simulink model "gm_hdl_model_fixed"  (R2024a)
settings: Solver=FixedStepDiscrete  StartTime=0.0  StopTime=SIM_TIME  RelTol=1e-3
model workspace (MAT data in the model file):
  HDLVAXIManagerConfig = hdlverifier.internal.AXIMaster.ConfigParams
undefined symbols (not defined in the file or in its folder): a, b, BUFFER_LEN, c, SAMPLING_FREQ, signal_1
libraries: hdlsllib x38, simulink_extras x4, simulink x2, dspsrcs4 x1, dsphdlxfrm2 x1
(part 1 of 3)
settings Model: SimulationMode=accelerator  Creator=Jan Rosa  LastModifiedBy=Jan Rosa
settings OptimizationCC: BlockReduction=off  ConditionallyExecuteInputs=off  DefaultParameterBehavior=Inlined  InheritOutputTypeSmallerThanSingle=on
settings DebuggingCC: SignalRangeChecking=warning  AlgebraicLoopMsg=error  SolverPrmCheckMsg=warning  InheritedTsInSrcMsg=none  SingleTaskRateTransMsg=error  UnderSpecifiedDataTypeMsg=warning  UnconnectedInputMsg=error  UnconnectedOutputMsg=error  UnconnectedLineMsg=error  ModelReferenceVersionMismatchMessage=warning  ModelReferenceIOMismatchMessage=warning  ModelReferenceNoExplicitFinalValueMsg=warning  StateNameClashWarn=warning
settings HardwareCC: ProdBitPerPointer=32  ProdBitPerSizeT=32  ProdBitPerPtrDiffT=32  ProdLargestAtomicFloat=None  ProdIntDivRoundTo=Undefined  ProdEndianess=Unspecified  ProdWordSize=32  ProdHWDeviceType=ASIC/FPGA->ASIC/FPGA  TargetBitPerPointer=64  TargetBitPerSizeT=64  TargetBitPerPtrDiffT=64  TargetLongLongMode=on  TargetIntDivRoundTo=Zero  TargetEndianess=LittleEndian  TargetWordSize=64  TargetHWDeviceType=Custom Processor->MATLAB Host Computer  ProdEqTarget=off
settings ModelReferenceCC: EnableRefExpFcnMdlSchedulingChecks=on  EnableParallelModelReferenceBuilds=on

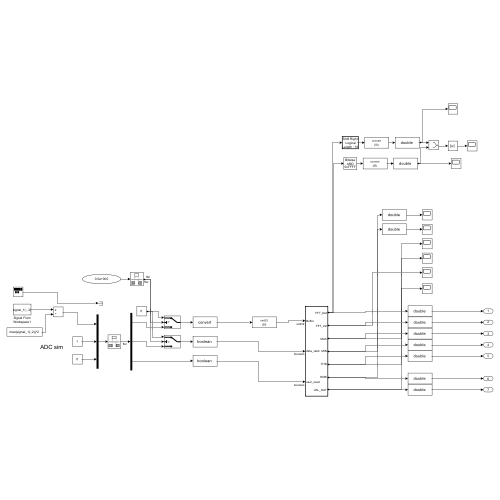
[thumbnail: Simulink's stored preview of the top-level diagram]
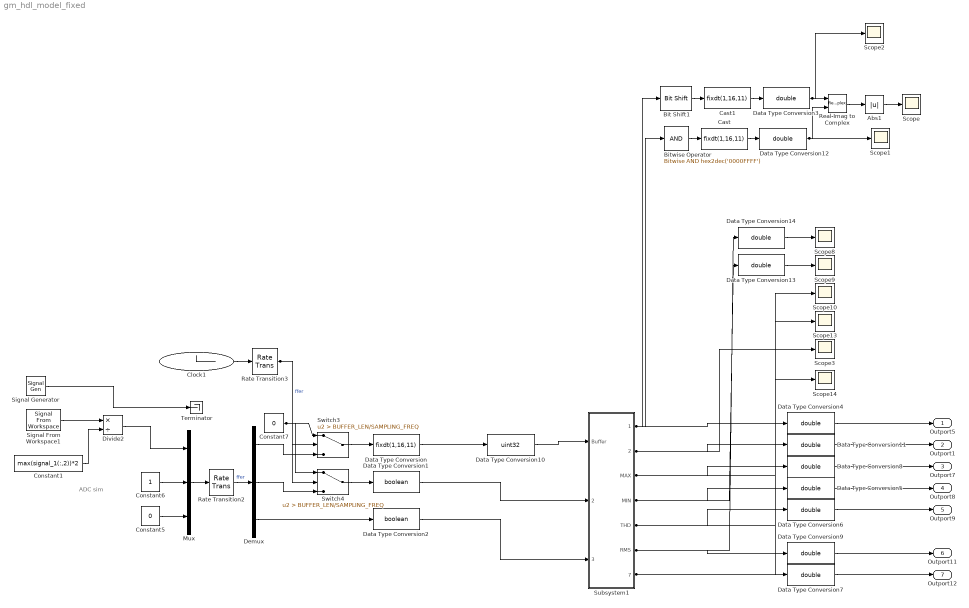
== system gm_hdl_model_fixed ==
  note: ADC sim
  Abs1 : Abs  SaturateOnIntegerOverflow=off
  Bit Shift1 : hdlsllib/Logic and Bit Operations/Bit Shift  mode=Shift Right Logical  N=16
  Bitwise Operator : simulink/Logic and Bit Operations/Bitwise Operator  logicop=AND  UseBitMask=on  BitMask=hex2dec('0000FFFF')  BitMaskRealWorld=Stored Integer
  Cast : DataTypeConversion  OutDataTypeStr=fixdt(1,16,11)  ConvertRealWorld=Stored Integer (SI)  SaturateOnIntegerOverflow=off  RndMeth=Floor
  Cast1 : DataTypeConversion  OutDataTypeStr=fixdt(1,16,11)  ConvertRealWorld=Stored Integer (SI)  SaturateOnIntegerOverflow=off  RndMeth=Floor
  Clock1 : Clock
  Constant1 : Constant  Value=max(signal_1(:,2))*2
  Constant5 : Constant  Value=0
  Constant6 : Constant
  Constant7 : Constant  Value=0  SampleTime=1/SAMPLING_FREQ
  Data Type Conversion : DataTypeConversion  OutDataTypeStr=fixdt(1,16,11)  SaturateOnIntegerOverflow=off  RndMeth=Floor  LockScale=on
  Data Type Conversion1 : DataTypeConversion  OutDataTypeStr=boolean  SaturateOnIntegerOverflow=off  RndMeth=Floor  LockScale=on
  Data Type Conversion10 : DataTypeConversion  OutDataTypeStr=uint32  ConvertRealWorld=Stored Integer (SI)  SaturateOnIntegerOverflow=off  RndMeth=Floor
  Data Type Conversion{3..9,11..14} (11 alike) : DataTypeConversion  OutDataTypeStr=double  SaturateOnIntegerOverflow=off  RndMeth=Floor
  Data Type Conversion2 : DataTypeConversion  OutDataTypeStr=boolean  SaturateOnIntegerOverflow=off  RndMeth=Floor  LockScale=on
  Demux : Demux  Outputs=3
  Divide2 : Product  Inputs=*/
  Mux : Mux  Inputs=3
  Rate Transition2 : RateTransition  Integrity=off  Deterministic=off  OutPortSampleTime=1/SAMPLING_FREQ
  Rate Transition3 : RateTransition  Integrity=off  Deterministic=off  OutPortSampleTime=1/SAMPLING_FREQ
  Real-Imag to Complex : RealImagToComplex
  Scope{,1..3,8..10,13..14} (9 alike) : Scope
  Signal Generator : SignalGenerator  WaveForm=square  Amplitude=0.49999  Frequency=SAMPLING_FREQ/(16*16)
  Signal From Workspace1 : dspsrcs4/Signal From Workspace  X=signal_1(:, 2)  Ts=1/SAMPLING_FREQ  nsamps=1  OutputAfterFinalValue=Cyclic repetition  ignoreOrWarnInputAndFrameLengths=off  OutputFrames=off
  Subsystem1 : Subsystem  TreatAsAtomicUnit=on
  Switch3 : Switch  Criteria=u2 > Threshold  Threshold=BUFFER_LEN/SAMPLING_FREQ  SaturateOnIntegerOverflow=off  InputSameDT=off
  Switch4 : Switch  Criteria=u2 > Threshold  Threshold=BUFFER_LEN/SAMPLING_FREQ  SaturateOnIntegerOverflow=off  InputSameDT=off
  Terminator : Terminator
  Outport5 : Outport
  Outport1 : Outport  Port=2
  Outport7 : Outport  Port=3
  Outport8 : Outport  Port=4
  Outport9 : Outport  Port=5
  Outport11 : Outport  Port=6
  Outport12 : Outport  Port=7
  wires:
  Data Type Conversion10/1 -> Subsystem1/1(Buffer)
  Signal Generator/1 -> Terminator/1
  Divide2/1 -> Mux/1
  Subsystem1/2(FFT_Val) -> Data Type Conversion11/1, Scope3/1
  Data Type Conversion/1 -> Data Type Conversion10/1
  Data Type Conversion1/1 -> Subsystem1/2(data_valid)
  Data Type Conversion2/1 -> Subsystem1/3(user_reset)
  Switch4/1 -> Data Type Conversion1/1
  Data Type Conversion13/1 -> Scope9/1
  Data Type Conversion14/1 -> Scope8/1
  Cast1/1 -> Data Type Conversion3/1
  Cast/1 -> Data Type Conversion12/1
  Data Type Conversion12/1 -> Real-Imag to Complex/2, Scope1/1
  Bitwise Operator/1 -> Cast/1
  Bit Shift1/1 -> Cast1/1
  Real-Imag to Complex/1 -> Abs1/1
  Data Type Conversion3/1 -> Real-Imag to Complex/1, Scope2/1
  Data Type Conversion11/1 -> Outport1/1
  Data Type Conversion9/1 -> Outport11/1
  Data Type Conversion7/1 -> Outport12/1
  Data Type Conversion6/1 -> Outport9/1
  Data Type Conversion5/1 -> Outport8/1
  Data Type Conversion8/1 -> Outport7/1
  Data Type Conversion4/1 -> Outport5/1
  Subsystem1/6(RMS) -> Data Type Conversion14/1, Data Type Conversion9/1
  Constant1/1 -> Divide2/2
  Constant6/1 -> Mux/2
  Signal From Workspace1/1 -> Divide2/1
  Constant5/1 -> Mux/3
  Rate Transition2/1 -> Demux/1  "ffer"
  Abs1/1 -> Scope/1
  Subsystem1/4(MIN) -> Data Type Conversion13/1, Data Type Conversion5/1
  Mux/1 -> Rate Transition2/1
  Demux/1 -> Switch3/3
  Switch3/1 -> Data Type Conversion/1
  Subsystem1/5(THD) -> Scope13/1, Data Type Conversion6/1
  Demux/3 -> Data Type Conversion2/1
  Clock1/1 -> Rate Transition3/1
  Demux/2 -> Switch4/3
  Subsystem1/3(MAX) -> Scope10/1, Data Type Conversion8/1
  Subsystem1/7(VAL_OUT) -> Scope14/1, Data Type Conversion7/1
  Rate Transition3/1 -> Switch3/2, Switch4/2  "ffer"
  Constant7/1 -> Switch3/1, Switch4/1
  Subsystem1/1(FFT_Dat) -> Bit Shift1/1, Bitwise Operator/1, Data Type Conversion4/1

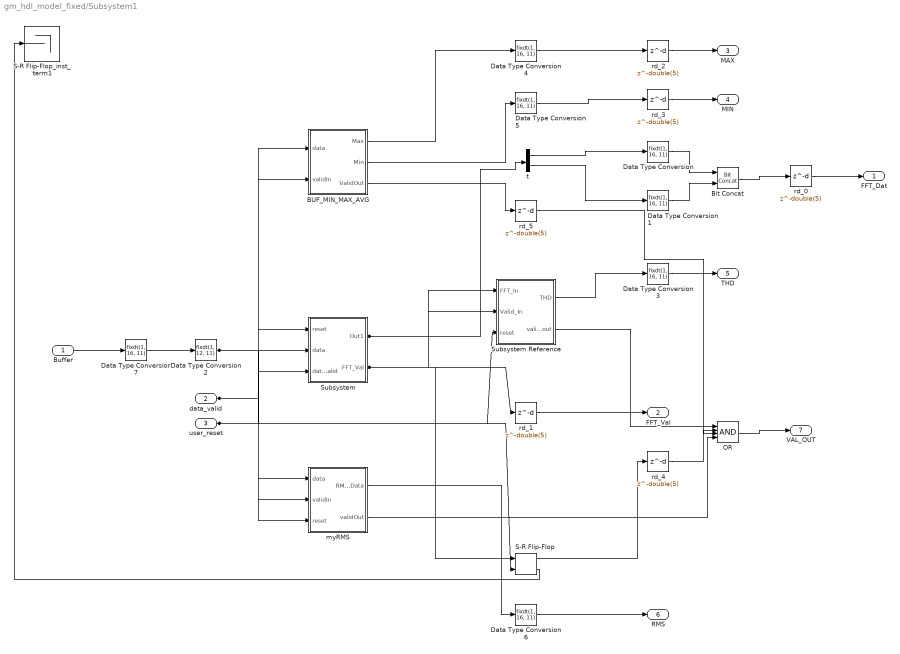
== system gm_hdl_model_fixed/Subsystem1 ==
  Buffer : Inport  OutDataTypeStr=uint32  PortDimensions=1  SampleTime=1e-08
  data_valid : Inport  Port=2  OutDataTypeStr=boolean  PortDimensions=1  SampleTime=1e-08
  user_reset : Inport  Port=3  OutDataTypeStr=boolean  PortDimensions=1  SampleTime=1e-08
  BUF_MIN_MAX_AVG : Subsystem
  Bit Concat : hdlsllib/Logic and Bit Operations/Bit Concat  numInputs=2
  Data Type Conversion{,1,3..6} (6 alike) : DataTypeConversion  OutDataTypeStr=fixdt(1, 16, 11)  SampleTime=1e-08  SaturateOnIntegerOverflow=off  RndMeth=Floor
  Data Type Conversion2 : DataTypeConversion  OutDataTypeStr=fixdt(1, 12, 11)  SampleTime=1e-08  SaturateOnIntegerOverflow=off  RndMeth=Floor
  Data Type Conversion7 : DataTypeConversion  OutDataTypeStr=fixdt(1, 16, 11)  ConvertRealWorld=Stored Integer (SI)  SampleTime=1e-08  SaturateOnIntegerOverflow=off  RndMeth=Floor
  OR : Logic  Inputs=4  AllPortsSameDT=off  OutDataTypeStr=boolean  SampleTime=1e-08
  S-R Flip-Flop : simulink_extras/Flip Flops/S-R Flip-Flop  initial_condition=0
  S-R Flip-Flop_inst_term1 : Terminator
  Subsystem : Subsystem
  Subsystem Reference : Subsystem
  myRMS : Subsystem
  rd_{0..5} (6 alike) : Delay  DelayLength=double(5)  InitialCondition=0  SampleTime=1e-08
  t : Demux  Outputs=2
  FFT_Dat : Outport  SampleTime=1e-08
  FFT_Val : Outport  Port=2  SampleTime=1e-08
  MAX : Outport  Port=3  SampleTime=1e-08
  MIN : Outport  Port=4  SampleTime=1e-08
  THD : Outport  Port=5  SampleTime=1e-08
  RMS : Outport  Port=6  SampleTime=1e-08
  VAL_OUT : Outport  Port=7  SampleTime=1e-08
  wires:
  Buffer/1 -> Data Type Conversion7/1
  data_valid/1 -> Subsystem/3(data_valid), myRMS/2(validIn), BUF_MIN_MAX_AVG/2(validIn)
  user_reset/1 -> Subsystem Reference/3(reset), Subsystem/1(reset), myRMS/3(reset), S-R Flip-Flop/2
  BUF_MIN_MAX_AVG/1(Max) -> Data Type Conversion4/1
  BUF_MIN_MAX_AVG/2(Min) -> Data Type Conversion5/1
  Data Type Conversion/1 -> Bit Concat/1
  Data Type Conversion1/1 -> Bit Concat/2
  Data Type Conversion2/1 -> Subsystem/2(data), BUF_MIN_MAX_AVG/1(data), myRMS/1(data)
  Data Type Conversion3/1 -> THD/1
  Data Type Conversion6/1 -> RMS/1
  Data Type Conversion7/1 -> Data Type Conversion2/1
  OR/1 -> VAL_OUT/1
  S-R Flip-Flop/2 -> S-R Flip-Flop_inst_term1/1
  Subsystem/1(Out1) -> t/1, Subsystem Reference/1(FFT_In)
  Subsystem Reference/1(THD) -> Data Type Conversion3/1
  Subsystem Reference/2(valid_out) -> OR/1
  myRMS/1(RMS_Data) -> Data Type Conversion6/1
  myRMS/2(validOut) -> OR/4
  t/1 -> Data Type Conversion/1
  t/2 -> Data Type Conversion1/1
  S-R Flip-Flop/1 -> rd_4/1
  BUF_MIN_MAX_AVG/3(ValidOut) -> rd_5/1
  Bit Concat/1 -> rd_0/1
  Subsystem/2(FFT_Val) -> rd_1/1, Subsystem Reference/2(Valid_In), S-R Flip-Flop/1
  Data Type Conversion4/1 -> rd_2/1
  Data Type Conversion5/1 -> rd_3/1
  rd_5/1 -> OR/3
  rd_1/1 -> FFT_Val/1
  rd_0/1 -> FFT_Dat/1
  rd_2/1 -> MAX/1
  rd_3/1 -> MIN/1
  rd_4/1 -> OR/2

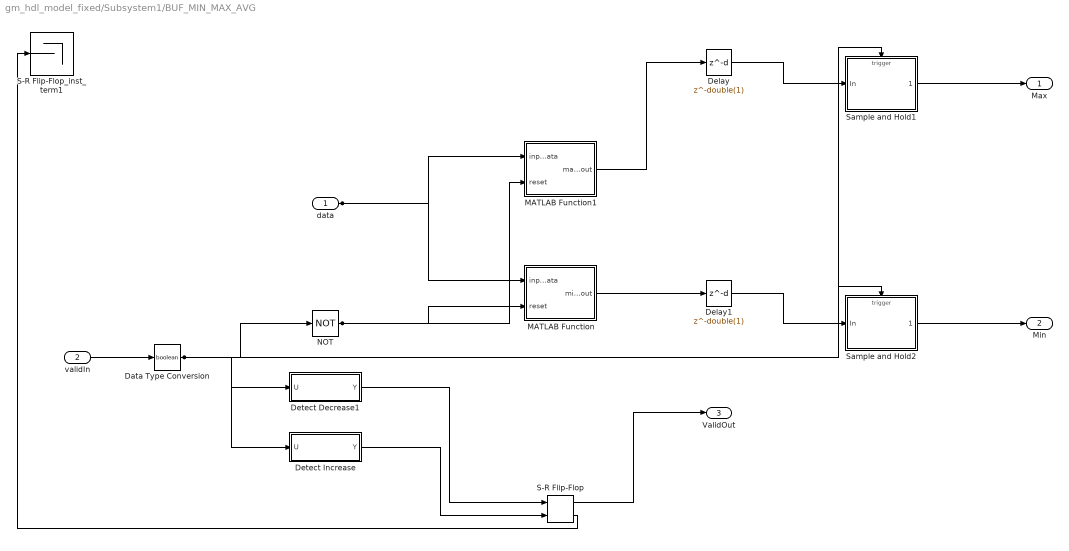
== system gm_hdl_model_fixed/Subsystem1/BUF_MIN_MAX_AVG ==
  data : Inport  OutDataTypeStr=fixdt(1, 12, 11)  PortDimensions=1  SampleTime=1e-08
  validIn : Inport  Port=2  OutDataTypeStr=boolean  PortDimensions=1  SampleTime=1e-08
  Data Type Conversion : DataTypeConversion  OutDataTypeStr=boolean
  Delay : Delay  DelayLength=double(1)  InitialCondition=0  SampleTime=1e-08
  Delay1 : Delay  DelayLength=double(1)  InitialCondition=0  SampleTime=1e-08
  Detect Decrease1 : Subsystem  mask(Detect Decrease){vinit=double(0), InputProcessing=Elements as channels (sample based), OutDataTypeStr=boolean}
      mask prompts: vinit "Simulink:masks:InitialCondition_MP"; InputProcessing "Simulink:masks:InputProcessing_MP"; OutDataTypeStr "Simulink:masks:OutputDataType_MP"
      mask help: Simulink:masks:DetectDecrease_MD
      mask init:
      | InputProcessing = 'Elements as channels (sample based)';
      | OutDataTypeStr = 'boolean';
      | vinit = double(0);
      mask TypeOptions InputProcessing: Simulink:masks:ColumnsAsChannelsFrameBased | Simulink:masks:ElementsAsChannelsSampleBased
      mask TypeOptions OutDataTypeStr: Simulink:masks:uint8 | Simulink:masks:boolean
      mask Display: fprintf('U < U/z')
  Detect Increase : Subsystem  mask(Detect Increase){vinit=double(0), InputProcessing=Elements as channels (sample based), OutDataTypeStr=boolean}
      mask prompts: vinit "Simulink:masks:InitialCondition_MP"; InputProcessing "Simulink:masks:InputProcessing_MP"; OutDataTypeStr "Simulink:masks:OutputDataType_MP"
      mask help: Simulink:masks:DetectIncrease_MD
      mask init:
      | InputProcessing = 'Elements as channels (sample based)';
      | OutDataTypeStr = 'boolean';
      | vinit = double(0);
      mask TypeOptions InputProcessing: Simulink:masks:ColumnsAsChannelsFrameBased | Simulink:masks:ElementsAsChannelsSampleBased
      mask TypeOptions OutDataTypeStr: Simulink:masks:uint8 | Simulink:masks:boolean
      mask Display: fprintf('U > U/z')
  MATLAB Function : Subsystem
  MATLAB Function1 : Subsystem
  NOT : Logic  Operator=NOT  Inputs=1  AllPortsSameDT=off  OutDataTypeStr=boolean  SampleTime=1e-08
  S-R Flip-Flop : simulink_extras/Flip Flops/S-R Flip-Flop  initial_condition=0
  S-R Flip-Flop_inst_term1 : Terminator
  Sample and Hold1 : Subsystem  mask(Sample and Hold){trig=Falling edge, initCond=double(0), latchinput=off}
      mask prompts: trig "dsp:DSPSignalOperationsBlockDialog:TriggerType_MP"; initCond "dsp:DSPSignalOperationsBlockDialog:InitialCondition_MP"; latchinput "dsp:DSPSignalOperationsBlockDialog:LatchInput_MP"
      mask help: dsp:DSPSignalOperationsBlockDialog:SampleAndHold_MaskDesc
      mask init:
      | initCond = double(0);
      | latchinput = double(0);
      | s = 'falling';
      | trig = double(2);
      mask Help: eval('blocksethelp');
      mask TypeOptions trig: dsp:DSPSignalOperationsBlockDialog:RisingEdge_MP | dsp:DSPSignalOperationsBlockDialog:FallingEdge_MP | dsp:DSPSignalOperationsBlockDialog:EitherEdge_MP
      mask Display: disp('S/H')
  Sample and Hold2 : Subsystem  mask(Sample and Hold){trig=Falling edge, initCond=double(0), latchinput=off}
      mask prompts: trig "dsp:DSPSignalOperationsBlockDialog:TriggerType_MP"; initCond "dsp:DSPSignalOperationsBlockDialog:InitialCondition_MP"; latchinput "dsp:DSPSignalOperationsBlockDialog:LatchInput_MP"
      mask help: dsp:DSPSignalOperationsBlockDialog:SampleAndHold_MaskDesc
      mask init:
      | initCond = double(0);
      | latchinput = double(0);
      | s = 'falling';
      | trig = double(2);
      mask Help: eval('blocksethelp');
      mask TypeOptions trig: dsp:DSPSignalOperationsBlockDialog:RisingEdge_MP | dsp:DSPSignalOperationsBlockDialog:FallingEdge_MP | dsp:DSPSignalOperationsBlockDialog:EitherEdge_MP
      mask Display: disp('S/H')
  Max : Outport  SampleTime=1e-08
  Min : Outport  Port=2  SampleTime=1e-08
  ValidOut : Outport  Port=3  SampleTime=1e-08
  wires:
  data/1 -> MATLAB Function1/1(input_data), MATLAB Function/1(input_data)
  validIn/1 -> Data Type Conversion/1
  Data Type Conversion/1 -> NOT/1, Detect Increase/1(U), Detect Decrease1/1(U), Sample and Hold1/Trigger, Sample and Hold2/Trigger
  Delay/1 -> Sample and Hold1/1(In)
  Delay1/1 -> Sample and Hold2/1(In)
  Detect Decrease1/1(Y) -> S-R Flip-Flop/1
  Detect Increase/1(Y) -> S-R Flip-Flop/2
  MATLAB Function/1(min_out) -> Delay1/1
  MATLAB Function1/1(max_out) -> Delay/1
  NOT/1 -> MATLAB Function1/2(reset), MATLAB Function/2(reset)
  S-R Flip-Flop/1 -> ValidOut/1
  S-R Flip-Flop/2 -> S-R Flip-Flop_inst_term1/1
  Sample and Hold1/1(" ") -> Max/1
  Sample and Hold2/1(" ") -> Min/1

== system gm_hdl_model_fixed/Subsystem1/Subsystem ==
  note: Divide by FFT length shift
  reset : Inport  OutDataTypeStr=boolean  PortDimensions=1  SampleTime=1e-08
  data : Inport  Port=2  OutDataTypeStr=fixdt(1, 12, 11)  PortDimensions=1  SampleTime=1e-08
  data_valid : Inport  Port=3  OutDataTypeStr=boolean  PortDimensions=1  SampleTime=1e-08
  Bit Shift : hdlsllib/Logic and Bit Operations/Bit Shift  mode=Shift Right Arithmetic  N=double(11)
  Complex to Real-Imag : ComplexToRealImag  SampleTime=1e-08
  Data Type Conversion : DataTypeConversion  OutDataTypeStr=fixdt(1, 12, 11)  SampleTime=1e-08  SaturateOnIntegerOverflow=off  RndMeth=Floor
  FFT : dsphdlxfrm2/FFT  Architecture=Streaming Radix 2^2  FFTLengthSource=Property  FFTLength=BUFFER_LEN  FFTLengthMax=1024  ComplexMultiplication=Use 4 multipliers and 2 adders  BitReversedOutput=off  BitReversedInput=off  Normalize=off  SimulateUsing=Code generation  RoundingMethod=Floor  ResetInputPort=on  StartOutputPort=off  EndOutputPort=off
  mux : Mux  Inputs=2
  Out1 : Outport  SampleTime=1e-08
  FFT_Val : Outport  Port=2  SampleTime=1e-08
  wires:
  reset/1 -> FFT/3
  data/1 -> FFT/1
  data_valid/1 -> FFT/2
  Bit Shift/1 -> Data Type Conversion/1
  Complex to Real-Imag/1 -> mux/1
  Complex to Real-Imag/2 -> mux/2
  Data Type Conversion/1 -> Out1/1
  FFT/1 -> Complex to Real-Imag/1
  FFT/2 -> FFT_Val/1
  mux/1 -> Bit Shift/1

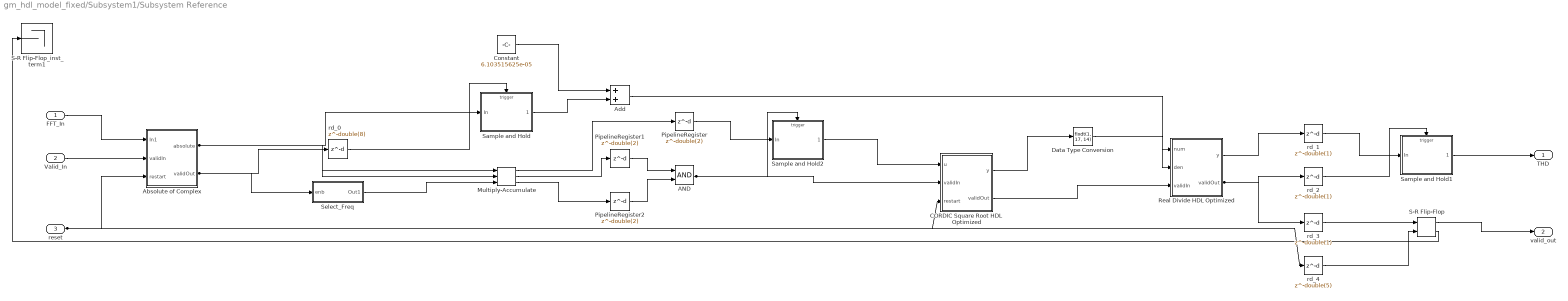
== system gm_hdl_model_fixed/Subsystem1/Subsystem Reference ==
  FFT_In : Inport  OutDataTypeStr=fixdt(1, 12, 11)  PortDimensions=[2]  SampleTime=1e-08
  Valid_In : Inport  Port=2  OutDataTypeStr=boolean  PortDimensions=1  SampleTime=1e-08
  reset : Inport  Port=3  OutDataTypeStr=boolean  PortDimensions=1  SampleTime=1e-08
  AND : Logic  AllPortsSameDT=off  OutDataTypeStr=boolean  SampleTime=1e-08
  Absolute of Complex : Subsystem
  Add : Sum  OutDataTypeStr=fixdt(1, 17, 14)  AccumDataTypeStr=fixdt(1, 17, 14)  SampleTime=1e-08
  CORDIC Square Root HDL Optimized : Subsystem  mask(CORDIC Square Root HDL Optimized){autoMaximumShiftVal=on, maximumShiftValue=double(10), nIterPerReg=double(1)}
      mask prompts: autoMaximumShiftVal "fixed:emblib:AutoCORDICMaxShiftValue"; maximumShiftValue "fixed:emblib:CORDICMaxShiftValue"; nIterPerReg "fixed:emblib:NumberOfIterationsPerReg"
      mask help: fixed:emblib:CORDICSquareRootHDLFullDescription
      mask Help: eval('embblk.embhelp(gcb)')
      mask Callback autoMaximumShiftVal:
      | autoMaxShiftVal = get_param(gcb,'autoMaximumShiftVal');
      | if strcmp(autoMaxShiftVal,'on')
      |     set_param(gcb,'MaskVisibilities',{'on','off','on'});
      | else
      |     set_param(gcb,'MaskVisibilities',{'on','on','on'});
      | end
      mask Display: disp('CORDIC Square Root\nHDL Optimized')
  Constant : Constant  Value=6.103515625e-05  OutDataTypeStr=fixdt(1, 16, 14)  SampleTime=1e-08
  Data Type Conversion : DataTypeConversion  OutDataTypeStr=fixdt(1, 17, 14)  SampleTime=1e-08  SaturateOnIntegerOverflow=off  RndMeth=Floor
  Multiply-Accumulate : hdlsllib/HDL Operations/Multiply-Accumulate  opMode=Streaming - using Number of Samples  initValueSetting=Dialog  initValue=0  initValueSetting2=Dialog  initValue2=0  initValueSetting3=Dialog  initValue3=0  num_samples=1015  RndMeth2=Floor  RndMeth3=Floor  datatype2=Inherit: Inherit via back propagation  datatype3=fixdt(1, 22, 20)  validOut=on  endInandOut=on  startOut=on  countOut=off  dim=-1  DoSatur=off  parallel=off
  PipelineRegister : Delay  DelayLength=double(2)  InitialCondition=0  SampleTime=1e-08
  PipelineRegister1 : Delay  DelayLength=double(2)  InitialCondition=0  SampleTime=1e-08
  PipelineRegister2 : Delay  DelayLength=double(2)  InitialCondition=0  SampleTime=1e-08
  Real Divide HDL Optimized : Subsystem  mask(Real Divide HDL Optimized){OutputType=fixdt(1,18,10)}
      mask prompts: OutputType "fixed:emblib:OutputPrototype"
      mask help: fixed:emblib:RealDivideFullDescription
      mask Help: eval('embblk.embhelp(gcb)')
      mask Display:
      | text(0.5,0.6,'den ~= 0','texmode','on','HorizontalAlignment','center')
      | text(0.5,0.4,'y = num/den','texmode','on','HorizontalAlignment','center')
  S-R Flip-Flop : simulink_extras/Flip Flops/S-R Flip-Flop  initial_condition=0
  S-R Flip-Flop_inst_term1 : Terminator
  Sample and Hold : Subsystem  mask(Sample and Hold){trig=Rising edge, initCond=double(0), latchinput=off}
      mask prompts: trig "dsp:DSPSignalOperationsBlockDialog:TriggerType_MP"; initCond "dsp:DSPSignalOperationsBlockDialog:InitialCondition_MP"; latchinput "dsp:DSPSignalOperationsBlockDialog:LatchInput_MP"
      mask help: dsp:DSPSignalOperationsBlockDialog:SampleAndHold_MaskDesc
      mask init:
      | initCond = double(0);
      | latchinput = double(0);
      | s = 'rising';
      | trig = double(1);
      mask Help: eval('blocksethelp');
      mask TypeOptions trig: dsp:DSPSignalOperationsBlockDialog:RisingEdge_MP | dsp:DSPSignalOperationsBlockDialog:FallingEdge_MP | dsp:DSPSignalOperationsBlockDialog:EitherEdge_MP
      mask Display: disp('S/H')
  Sample and Hold1 : Subsystem  mask(Sample and Hold){trig=Rising edge, initCond=double(0), latchinput=off}
      mask prompts: trig "dsp:DSPSignalOperationsBlockDialog:TriggerType_MP"; initCond "dsp:DSPSignalOperationsBlockDialog:InitialCondition_MP"; latchinput "dsp:DSPSignalOperationsBlockDialog:LatchInput_MP"
      mask help: dsp:DSPSignalOperationsBlockDialog:SampleAndHold_MaskDesc
      mask init:
      | initCond = double(0);
      | latchinput = double(0);
      | s = 'rising';
      | trig = double(1);
      mask Help: eval('blocksethelp');
      mask TypeOptions trig: dsp:DSPSignalOperationsBlockDialog:RisingEdge_MP | dsp:DSPSignalOperationsBlockDialog:FallingEdge_MP | dsp:DSPSignalOperationsBlockDialog:EitherEdge_MP
      mask Display: disp('S/H')
  Sample and Hold2 : Subsystem  mask(Sample and Hold){trig=Rising edge, initCond=double(0), latchinput=off}
      mask prompts: trig "dsp:DSPSignalOperationsBlockDialog:TriggerType_MP"; initCond "dsp:DSPSignalOperationsBlockDialog:InitialCondition_MP"; latchinput "dsp:DSPSignalOperationsBlockDialog:LatchInput_MP"
      mask help: dsp:DSPSignalOperationsBlockDialog:SampleAndHold_MaskDesc
      mask init:
      | initCond = double(0);
      | latchinput = double(0);
      | s = 'rising';
      | trig = double(1);
      mask Help: eval('blocksethelp');
      mask TypeOptions trig: dsp:DSPSignalOperationsBlockDialog:RisingEdge_MP | dsp:DSPSignalOperationsBlockDialog:FallingEdge_MP | dsp:DSPSignalOperationsBlockDialog:EitherEdge_MP
      mask Display: disp('S/H')
  Select_Freq : Subsystem
  rd_0 : Delay  DelayLength=double(8)  InitialCondition=0  SampleTime=1e-08
  rd_1 : Delay  DelayLength=double(1)  InitialCondition=0  SampleTime=1e-08
  rd_2 : Delay  DelayLength=double(1)  InitialCondition=0  SampleTime=1e-08
  rd_3 : Delay  DelayLength=double(1)  InitialCondition=0  SampleTime=1e-08
  rd_4 : Delay  DelayLength=double(5)  InitialCondition=0  SampleTime=1e-08
  THD : Outport  SampleTime=1e-08
  valid_out : Outport  Port=2  SampleTime=1e-08
  wires:
  FFT_In/1 -> Absolute of Complex/1(In1)
  Valid_In/1 -> Absolute of Complex/2(validIn)
  AND/1 -> CORDIC Square Root HDL Optimized/2(validIn), Sample and Hold2/Trigger
  Absolute of Complex/1(absolute) -> Multiply-Accumulate/2, Multiply-Accumulate/1, Sample and Hold/1(In)
  Absolute of Complex/2(validOut) -> rd_0/1, Select_Freq/1(enb)
  Add/1 -> Real Divide HDL Optimized/2(den)
  CORDIC Square Root HDL Optimized/1(y) -> Data Type Conversion/1
  CORDIC Square Root HDL Optimized/2(validOut) -> Real Divide HDL Optimized/3(validIn)
  Constant/1 -> Add/1
  Data Type Conversion/1 -> Real Divide HDL Optimized/1(num)
  PipelineRegister/1 -> Sample and Hold2/1(In)
  PipelineRegister1/1 -> AND/1
  PipelineRegister2/1 -> AND/2
  Real Divide HDL Optimized/1(y) -> rd_1/1
  Real Divide HDL Optimized/2(validOut) -> rd_3/1, rd_2/1
  S-R Flip-Flop/1 -> valid_out/1
  S-R Flip-Flop/2 -> S-R Flip-Flop_inst_term1/1
  Sample and Hold/1(" ") -> Add/2
  Sample and Hold1/1(" ") -> THD/1
  Sample and Hold2/1(" ") -> CORDIC Square Root HDL Optimized/1(u)
  Select_Freq/1(Out1) -> Multiply-Accumulate/3
  reset/1 -> rd_4/1, Absolute of Complex/3(restart), CORDIC Square Root HDL Optimized/3(restart)
  rd_4/1 -> S-R Flip-Flop/2
  rd_0/1 -> Sample and Hold/Trigger
  rd_1/1 -> Sample and Hold1/1(In)
  rd_2/1 -> Sample and Hold1/Trigger
  rd_3/1 -> S-R Flip-Flop/1
  Multiply-Accumulate/1 -> PipelineRegister/1
  Multiply-Accumulate/2 -> PipelineRegister1/1
  Multiply-Accumulate/3 -> PipelineRegister2/1

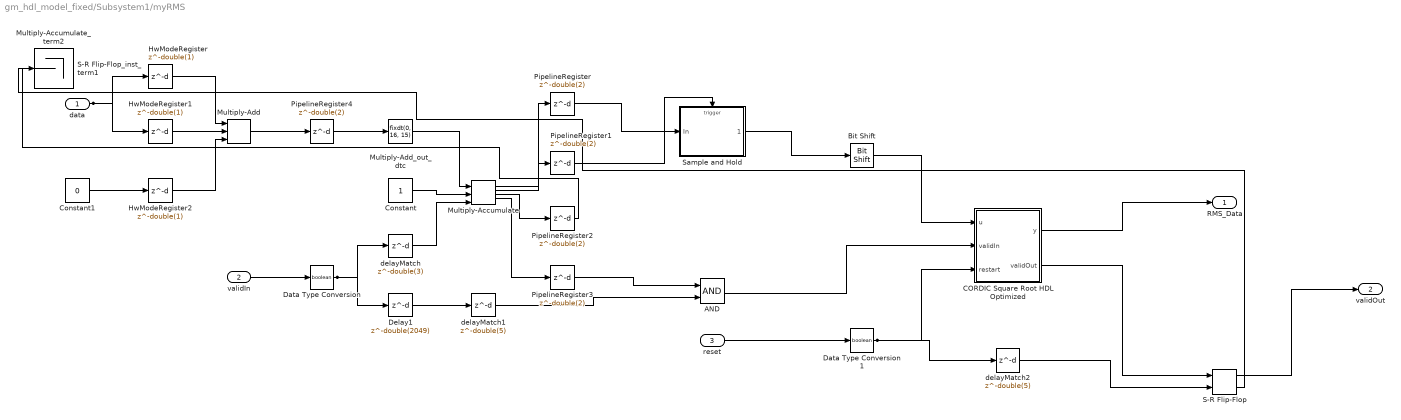
== system gm_hdl_model_fixed/Subsystem1/myRMS ==
  data : Inport  OutDataTypeStr=fixdt(1, 12, 11)  PortDimensions=1  SampleTime=1e-08
  validIn : Inport  Port=2  OutDataTypeStr=boolean  PortDimensions=1  SampleTime=1e-08
  reset : Inport  Port=3  OutDataTypeStr=boolean  PortDimensions=1  SampleTime=1e-08
  AND : Logic  AllPortsSameDT=off  OutDataTypeStr=boolean  SampleTime=1e-08
  Bit Shift : hdlsllib/Logic and Bit Operations/Bit Shift  mode=Shift Right Arithmetic  N=double(11)
  CORDIC Square Root HDL Optimized : Subsystem  mask(CORDIC Square Root HDL Optimized){autoMaximumShiftVal=on, maximumShiftValue=double(10), nIterPerReg=double(1)}
      mask prompts: autoMaximumShiftVal "fixed:emblib:AutoCORDICMaxShiftValue"; maximumShiftValue "fixed:emblib:CORDICMaxShiftValue"; nIterPerReg "fixed:emblib:NumberOfIterationsPerReg"
      mask help: fixed:emblib:CORDICSquareRootHDLFullDescription
      mask Help: eval('embblk.embhelp(gcb)')
      mask Callback autoMaximumShiftVal:
      | autoMaxShiftVal = get_param(gcb,'autoMaximumShiftVal');
      | if strcmp(autoMaxShiftVal,'on')
      |     set_param(gcb,'MaskVisibilities',{'on','off','on'});
      | else
      |     set_param(gcb,'MaskVisibilities',{'on','on','on'});
      | end
      mask Display: disp('CORDIC Square Root\nHDL Optimized')
  Constant : Constant  OutDataTypeStr=fixdt(0, 16, 15)  SampleTime=1e-08
  Constant1 : Constant  Value=0  OutDataTypeStr=fixdt(1, 12, 11)  SampleTime=1e-08
  Data Type Conversion : DataTypeConversion  OutDataTypeStr=boolean
  Data Type Conversion1 : DataTypeConversion  OutDataTypeStr=boolean
  Delay1 : Delay  DelayLength=double(2049)  InitialCondition=0  SampleTime=1e-08
  HwModeRegister : Delay  DelayLength=double(1)  InitialCondition=0  SampleTime=1e-08
  HwModeRegister1 : Delay  DelayLength=double(1)  InitialCondition=0  SampleTime=1e-08
  HwModeRegister2 : Delay  DelayLength=double(1)  InitialCondition=0  SampleTime=1e-08
  Multiply-Accumulate : hdlsllib/HDL Operations/Multiply-Accumulate  opMode=Streaming - using Number of Samples  initValueSetting=Dialog  initValue=0  initValueSetting2=Dialog  initValue2=0  initValueSetting3=Dialog  initValue3=0  num_samples=2048  RndMeth2=Floor  RndMeth3=Floor  datatype2=Inherit: Inherit via back propagation  datatype3=fixdt(0, 16, 7)  validOut=on  endInandOut=on  startOut=on  countOut=on  dim=-1  DoSatur=off  parallel=off
  Multiply-Accumulate_term2 : Terminator
  Multiply-Add : hdlsllib/HDL Operations/Multiply-Add  Function=c+(a.*b)  datatype=fixdt(1, 25, 22)  DoSatur=off  FMA=off
  Multiply-Add_out_dtc : DataTypeConversion  OutDataTypeStr=fixdt(0, 16, 15)  SampleTime=1e-08  SaturateOnIntegerOverflow=off  RndMeth=Floor
  PipelineRegister{,1,3..4} (4 alike) : Delay  DelayLength=double(2)  InitialCondition=0  SampleTime=1e-08
  PipelineRegister2 : Delay  DelayLength=double(2)  InitialCondition=1  SampleTime=1e-08
  S-R Flip-Flop : simulink_extras/Flip Flops/S-R Flip-Flop  initial_condition=0
  S-R Flip-Flop_inst_term1 : Terminator
  Sample and Hold : Subsystem  mask(Sample and Hold){trig=Rising edge, initCond=double(0), latchinput=off}
      mask prompts: trig "dsp:DSPSignalOperationsBlockDialog:TriggerType_MP"; initCond "dsp:DSPSignalOperationsBlockDialog:InitialCondition_MP"; latchinput "dsp:DSPSignalOperationsBlockDialog:LatchInput_MP"
      mask help: dsp:DSPSignalOperationsBlockDialog:SampleAndHold_MaskDesc
      mask init:
      | initCond = double(0);
      | latchinput = double(0);
      | s = 'rising';
      | trig = double(1);
      mask Help: eval('blocksethelp');
      mask TypeOptions trig: dsp:DSPSignalOperationsBlockDialog:RisingEdge_MP | dsp:DSPSignalOperationsBlockDialog:FallingEdge_MP | dsp:DSPSignalOperationsBlockDialog:EitherEdge_MP
      mask Display: disp('S/H')
  delayMatch : Delay  DelayLength=double(3)  InitialCondition=0  SampleTime=1e-08
  delayMatch1 : Delay  DelayLength=double(5)  InitialCondition=0  SampleTime=1e-08
  delayMatch2 : Delay  DelayLength=double(5)  InitialCondition=0  SampleTime=1e-08
  RMS_Data : Outport  SampleTime=1e-08
  validOut : Outport  Port=2  SampleTime=1e-08
  wires:
  data/1 -> HwModeRegister/1, HwModeRegister1/1
  validIn/1 -> Data Type Conversion/1
  reset/1 -> Data Type Conversion1/1
  AND/1 -> CORDIC Square Root HDL Optimized/2(validIn)
  Bit Shift/1 -> CORDIC Square Root HDL Optimized/1(u)
  CORDIC Square Root HDL Optimized/1(y) -> RMS_Data/1
  CORDIC Square Root HDL Optimized/2(validOut) -> S-R Flip-Flop/1
  Constant/1 -> Multiply-Accumulate/2
  Constant1/1 -> HwModeRegister2/1
  delayMatch/1 -> Multiply-Accumulate/3
  delayMatch2/1 -> S-R Flip-Flop/2
  delayMatch1/1 -> AND/2
  PipelineRegister/1 -> Sample and Hold/1(In)
  PipelineRegister1/1 -> Sample and Hold/Trigger
  PipelineRegister2/1 -> Multiply-Accumulate_term2/1
  PipelineRegister3/1 -> AND/1
  Multiply-Add_out_dtc/1 -> Multiply-Accumulate/1
  S-R Flip-Flop/1 -> validOut/1
  S-R Flip-Flop/2 -> S-R Flip-Flop_inst_term1/1
  Sample and Hold/1(" ") -> Bit Shift/1
  PipelineRegister4/1 -> Multiply-Add_out_dtc/1
  Data Type Conversion/1 -> delayMatch/1, Delay1/1
  Delay1/1 -> delayMatch1/1
  Data Type Conversion1/1 -> delayMatch2/1, CORDIC Square Root HDL Optimized/3(restart)
  Multiply-Accumulate/1 -> PipelineRegister/1
  Multiply-Accumulate/2 -> PipelineRegister1/1
  Multiply-Accumulate/3 -> PipelineRegister2/1
  Multiply-Accumulate/4 -> PipelineRegister3/1
  Multiply-Add/1 -> PipelineRegister4/1
  HwModeRegister/1 -> Multiply-Add/1
  HwModeRegister1/1 -> Multiply-Add/2
  HwModeRegister2/1 -> Multiply-Add/3

== system gm_hdl_model_fixed/Subsystem1/BUF_MIN_MAX_AVG/Detect Decrease1 ==
  note: U(k)
  note: Edge
  U : Inport  OutDataTypeStr=boolean  SampleTime=1e-08
  Delay Input1 : UnitDelay  SampleTime=1e-08
  FixPt Relational Operator : RelationalOperator  Operator=<  OutDataTypeStr=boolean  SampleTime=1e-08  InputSameDT=off
  Y : Outport  SampleTime=1e-08
  wires:
  U/1 -> FixPt Relational Operator/1, Delay Input1/1
  Delay Input1/1 -> FixPt Relational Operator/2
  FixPt Relational Operator/1 -> Y/1

== system gm_hdl_model_fixed/Subsystem1/BUF_MIN_MAX_AVG/Detect Increase ==
  note: U(k)
  note: Edge
  U : Inport  OutDataTypeStr=boolean  SampleTime=1e-08
  Delay Input1 : UnitDelay  SampleTime=1e-08
  FixPt Relational Operator : RelationalOperator  Operator=>  OutDataTypeStr=boolean  SampleTime=1e-08  InputSameDT=off
  Y : Outport  SampleTime=1e-08
  wires:
  U/1 -> FixPt Relational Operator/1, Delay Input1/1
  Delay Input1/1 -> FixPt Relational Operator/2
  FixPt Relational Operator/1 -> Y/1

== system gm_hdl_model_fixed/Subsystem1/BUF_MIN_MAX_AVG/MATLAB Function ==
  input_data : Inport  OutDataTypeStr=fixdt(1, 12, 11)  PortDimensions=1  SampleTime=1e-08
  reset : Inport  Port=2  OutDataTypeStr=boolean  PortDimensions=1  SampleTime=1e-08
  MATLAB Function : MATLAB Function  TreatAsAtomicUnit=on
  min_out : Outport  SampleTime=1e-08
  wires:
  MATLAB Function/1(min_out) -> min_out/1
  input_data/1 -> MATLAB Function/1(input_data)
  reset/1 -> MATLAB Function/2(reset)

== system gm_hdl_model_fixed/Subsystem1/BUF_MIN_MAX_AVG/MATLAB Function1 ==
  input_data : Inport  OutDataTypeStr=fixdt(1, 12, 11)  PortDimensions=1  SampleTime=1e-08
  reset : Inport  Port=2  OutDataTypeStr=boolean  PortDimensions=1  SampleTime=1e-08
  MATLAB Function1 : MATLAB Function  TreatAsAtomicUnit=on
  max_out : Outport  SampleTime=1e-08
  wires:
  MATLAB Function1/1(max_out) -> max_out/1
  input_data/1 -> MATLAB Function1/1(input_data)
  reset/1 -> MATLAB Function1/2(reset)

== system gm_hdl_model_fixed/Subsystem1/BUF_MIN_MAX_AVG/Sample and Hold1 ==
  In : Inport  OutDataTypeStr=fixdt(1, 12, 11)
  Trigger : TriggerPort  VariantControl=(inherit)  OutDataTypeStr=boolean
  " " : Outport  InitialOutput=0
  wires:
  In/1 -> " "/1

== system gm_hdl_model_fixed/Subsystem1/BUF_MIN_MAX_AVG/Sample and Hold2 ==
  In : Inport  OutDataTypeStr=fixdt(1, 12, 11)
  Trigger : TriggerPort  VariantControl=(inherit)  OutDataTypeStr=boolean
  " " : Outport  InitialOutput=0
  wires:
  In/1 -> " "/1

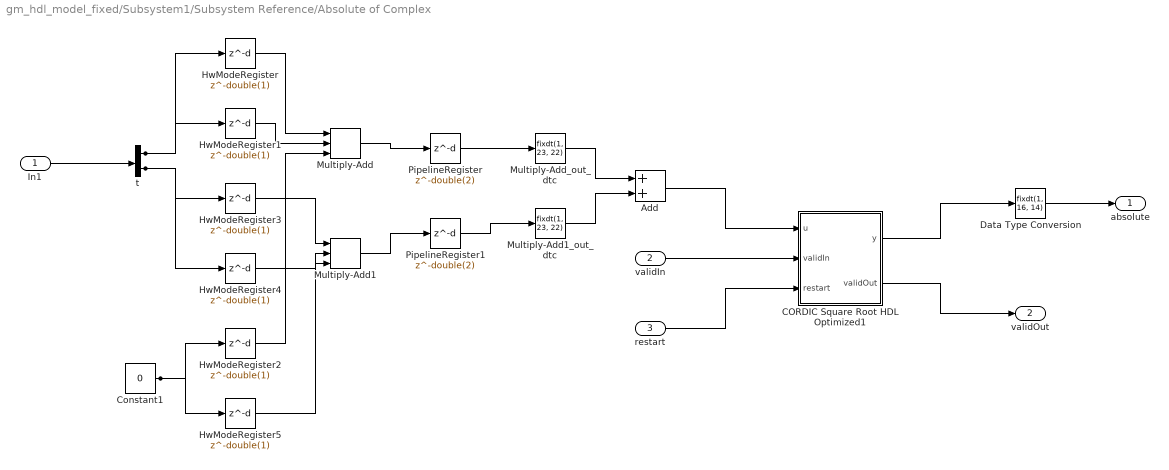
== system gm_hdl_model_fixed/Subsystem1/Subsystem Reference/Absolute of Complex ==
  In1 : Inport  OutDataTypeStr=fixdt(1, 12, 11)  PortDimensions=[2]  SampleTime=1e-08
  validIn : Inport  Port=2  OutDataTypeStr=boolean  PortDimensions=1  SampleTime=1e-08
  restart : Inport  Port=3  OutDataTypeStr=boolean  PortDimensions=1  SampleTime=1e-08
  Add : Sum  OutDataTypeStr=fixdt(1, 24, 22)  AccumDataTypeStr=fixdt(1, 24, 22)  SampleTime=1e-08
  CORDIC Square Root HDL Optimized1 : Subsystem  mask(CORDIC Square Root HDL Optimized){autoMaximumShiftVal=on, maximumShiftValue=double(10), nIterPerReg=double(1)}
      mask prompts: autoMaximumShiftVal "fixed:emblib:AutoCORDICMaxShiftValue"; maximumShiftValue "fixed:emblib:CORDICMaxShiftValue"; nIterPerReg "fixed:emblib:NumberOfIterationsPerReg"
      mask help: fixed:emblib:CORDICSquareRootHDLFullDescription
      mask Help: eval('embblk.embhelp(gcb)')
      mask Callback autoMaximumShiftVal:
      | autoMaxShiftVal = get_param(gcb,'autoMaximumShiftVal');
      | if strcmp(autoMaxShiftVal,'on')
      |     set_param(gcb,'MaskVisibilities',{'on','off','on'});
      | else
      |     set_param(gcb,'MaskVisibilities',{'on','on','on'});
      | end
      mask Display: disp('CORDIC Square Root\nHDL Optimized')
  Constant1 : Constant  Value=0  OutDataTypeStr=fixdt(1, 12, 11)  SampleTime=1e-08
  Data Type Conversion : DataTypeConversion  OutDataTypeStr=fixdt(1, 16, 14)  SampleTime=1e-08  SaturateOnIntegerOverflow=off  RndMeth=Floor
  HwModeRegister{,1..5} (6 alike) : Delay  DelayLength=double(1)  InitialCondition=0  SampleTime=1e-08
  Multiply-Add : hdlsllib/HDL Operations/Multiply-Add  Function=c+(a.*b)  datatype=fixdt(1, 25, 22)  DoSatur=off  FMA=off
  Multiply-Add1 : hdlsllib/HDL Operations/Multiply-Add  Function=c+(a.*b)  datatype=fixdt(1, 25, 22)  DoSatur=off  FMA=off
  Multiply-Add1_out_dtc : DataTypeConversion  OutDataTypeStr=fixdt(1, 23, 22)  SampleTime=1e-08  SaturateOnIntegerOverflow=off  RndMeth=Floor
  Multiply-Add_out_dtc : DataTypeConversion  OutDataTypeStr=fixdt(1, 23, 22)  SampleTime=1e-08  SaturateOnIntegerOverflow=off  RndMeth=Floor
  PipelineRegister : Delay  DelayLength=double(2)  InitialCondition=0  SampleTime=1e-08
  PipelineRegister1 : Delay  DelayLength=double(2)  InitialCondition=0  SampleTime=1e-08
  t : Demux  Outputs=2
  absolute : Outport  SampleTime=1e-08
  validOut : Outport  Port=2  SampleTime=1e-08
  wires:
  In1/1 -> t/1
  validIn/1 -> CORDIC Square Root HDL Optimized1/2(validIn)
  restart/1 -> CORDIC Square Root HDL Optimized1/3(restart)
  Add/1 -> CORDIC Square Root HDL Optimized1/1(u)
  CORDIC Square Root HDL Optimized1/1(y) -> Data Type Conversion/1
  CORDIC Square Root HDL Optimized1/2(validOut) -> validOut/1
  Constant1/1 -> HwModeRegister2/1, HwModeRegister5/1
  Data Type Conversion/1 -> absolute/1
  Multiply-Add_out_dtc/1 -> Add/1
  Multiply-Add1_out_dtc/1 -> Add/2
  t/1 -> HwModeRegister/1, HwModeRegister1/1
  t/2 -> HwModeRegister3/1, HwModeRegister4/1
  PipelineRegister/1 -> Multiply-Add_out_dtc/1
  PipelineRegister1/1 -> Multiply-Add1_out_dtc/1
  Multiply-Add/1 -> PipelineRegister/1
  HwModeRegister/1 -> Multiply-Add/1
  HwModeRegister1/1 -> Multiply-Add/2
  HwModeRegister2/1 -> Multiply-Add/3
  Multiply-Add1/1 -> PipelineRegister1/1
  HwModeRegister3/1 -> Multiply-Add1/1
  HwModeRegister4/1 -> Multiply-Add1/2
  HwModeRegister5/1 -> Multiply-Add1/3

== system gm_hdl_model_fixed/Subsystem1/Subsystem Reference/CORDIC Square Root HDL Optimized ==
  u : Inport  OutDataTypeStr=fixdt(1, 22, 20)  SampleTime=1e-08
  validIn : Inport  Port=2  OutDataTypeStr=boolean  SampleTime=1e-08
  restart : Inport  Port=3  OutDataTypeStr=boolean  SampleTime=1e-08
  Bit Shift Arithmetic : Subsystem
  Cast to Union of Types : Subsystem
  Data Type Conversion : DataTypeConversion  OutDataTypeStr=fixdt(1,22,20)
  Synchronous Subsystem : Subsystem
  y : Outport  SampleTime=1e-08
  validOut : Outport  Port=2  SampleTime=1e-08
  wires:
  u/1 -> Cast to Union of Types/1(Xref), Synchronous Subsystem/1(u)
  validIn/1 -> Synchronous Subsystem/2(validIn)
  restart/1 -> Synchronous Subsystem/3(restart)
  Bit Shift Arithmetic/1(y) -> Data Type Conversion/1
  Cast to Union of Types/1(Cout) -> Bit Shift Arithmetic/1(u)
  Data Type Conversion/1 -> y/1
  Synchronous Subsystem/1(dataOut) -> Cast to Union of Types/2(Cin)
  Synchronous Subsystem/2(eOut) -> Bit Shift Arithmetic/2(e)
  Synchronous Subsystem/3(isZero) -> Bit Shift Arithmetic/3(isZero)
  Synchronous Subsystem/4(validOut) -> validOut/1

== system gm_hdl_model_fixed/Subsystem1/Subsystem Reference/Real Divide HDL Optimized ==
  num : Inport  OutDataTypeStr=fixdt(1, 17, 14)  SampleTime=1e-08
  den : Inport  Port=2  OutDataTypeStr=fixdt(1, 17, 14)  SampleTime=1e-08
  validIn : Inport  Port=3  OutDataTypeStr=boolean  SampleTime=1e-08
  ForEach - Real Divide_instance1 : Subsystem
  Reshape to original size : Subsystem
  Verify divide sizes : Subsystem
  rd_0 : Delay  DelayLength=double(4)  InitialCondition=0  SampleTime=1e-08
  y = u(1) : Subsystem
  y : Outport  SampleTime=1e-08
  validOut : Outport  Port=2  SampleTime=1e-08
  wires:
  num/1 -> Verify divide sizes/2(numerator), Reshape to original size/2(u)
  den/1 -> Verify divide sizes/1(denominator)
  validIn/1 -> ForEach - Real Divide_instance1/3(validIn)
  ForEach - Real Divide_instance1/1(y) -> Reshape to original size/1(y)
  ForEach - Real Divide_instance1/2(validOut) -> rd_0/1
  Reshape to original size/1(z) -> y/1
  Verify divide sizes/1(den) -> ForEach - Real Divide_instance1/1(den)
  Verify divide sizes/2(num) -> ForEach - Real Divide_instance1/2(num)
  y = u(1)/1(y) -> validOut/1
  rd_0/1 -> y = u(1)/1(u)

== system gm_hdl_model_fixed/Subsystem1/Subsystem Reference/Sample and Hold ==
  In : Inport  OutDataTypeStr=fixdt(1, 16, 14)
  Trigger : TriggerPort  VariantControl=(inherit)  OutDataTypeStr=boolean
  " " : Outport  InitialOutput=0
  wires:
  In/1 -> " "/1

== system gm_hdl_model_fixed/Subsystem1/Subsystem Reference/Sample and Hold1 ==
  In : Inport  OutDataTypeStr=fixdt(1, 18, 10)
  Trigger : TriggerPort  VariantControl=(inherit)  OutDataTypeStr=boolean
  " " : Outport  InitialOutput=0
  wires:
  In/1 -> " "/1

== system gm_hdl_model_fixed/Subsystem1/Subsystem Reference/Sample and Hold2 ==
  In : Inport  OutDataTypeStr=fixdt(1, 22, 20)
  Trigger : TriggerPort  VariantControl=(inherit)  OutDataTypeStr=boolean
  " " : Outport  InitialOutput=0
  wires:
  In/1 -> " "/1

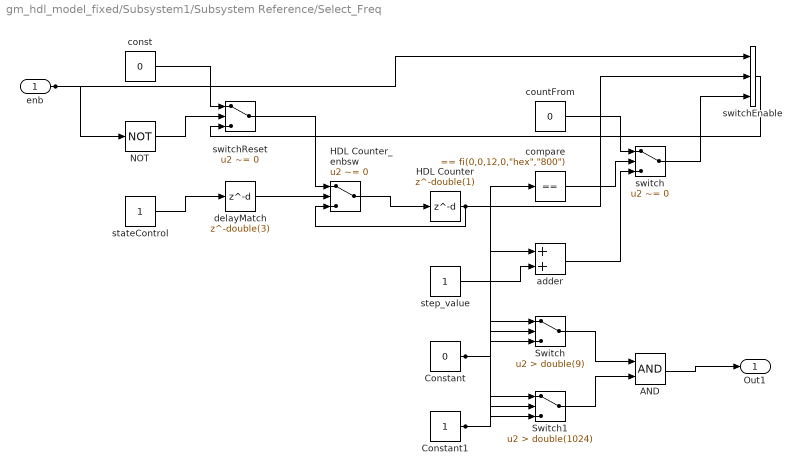
== system gm_hdl_model_fixed/Subsystem1/Subsystem Reference/Select_Freq ==
  enb : Inport  OutDataTypeStr=boolean  PortDimensions=1  SampleTime=1e-08
  AND : Logic  AllPortsSameDT=off  OutDataTypeStr=boolean  SampleTime=1e-08
  Constant : Constant  Value=0  OutDataTypeStr=boolean  SampleTime=1e-08
  Constant1 : Constant  OutDataTypeStr=boolean  SampleTime=1e-08
  HDL Counter : Delay  DelayLength=double(1)  InitialCondition=0  SampleTime=1e-08
  HDL Counter_enbsw : Switch  Criteria=u2 ~= 0  Threshold=double(0)  OutDataTypeStr=fixdt(0, 12, 0)  SampleTime=1e-08  SaturateOnIntegerOverflow=off  InputSameDT=off
  NOT : Logic  Operator=NOT  Inputs=1  AllPortsSameDT=off  OutDataTypeStr=boolean  SampleTime=1e-08
  Switch : Switch  Criteria=u2 > Threshold  Threshold=double(9)  OutDataTypeStr=boolean  SampleTime=1e-08  SaturateOnIntegerOverflow=off  InputSameDT=off
  Switch1 : Switch  Criteria=u2 > Threshold  Threshold=double(1024)  OutDataTypeStr=boolean  SampleTime=1e-08  SaturateOnIntegerOverflow=off  InputSameDT=off
  adder : Sum  OutDataTypeStr=fixdt(0, 12, 0)  AccumDataTypeStr=fixdt(0, 12, 0)  SampleTime=1e-08
  compare : simulink/Logic and Bit Operations/Compare To Constant  relop===  const="fi(0,0,12,0,\"hex\",\"800\")"  OutDataTypeStr=boolean
  const : Constant  Value=0  VectorParams1D=off  OutDataTypeStr=fixdt(0, 12, 0)  SampleTime=1e-08
  countFrom : Constant  Value=0  VectorParams1D=off  OutDataTypeStr=fixdt(0, 12, 0)  SampleTime=1e-08
  delayMatch : Delay  DelayLength=double(3)  InitialCondition=0  SampleTime=1e-08
  stateControl : Constant  OutDataTypeStr=boolean  SampleTime=1e-08
  step_value : Constant  VectorParams1D=off  OutDataTypeStr=fixdt(0, 12, 0)  SampleTime=1e-08
  switch : Switch  Criteria=u2 ~= 0  Threshold=double(0)  OutDataTypeStr=fixdt(0, 12, 0)  SampleTime=1e-08  SaturateOnIntegerOverflow=off  InputSameDT=off
  switchEnable : MultiPortSwitch  DataPortOrder=Zero-based contiguous  Inputs=2  DiagnosticForDefault=None  zeroidx=on  OutDataTypeStr=fixdt(0, 12, 0)  SampleTime=1e-08  SaturateOnIntegerOverflow=off  InputSameDT=off
  switchReset : Switch  Criteria=u2 ~= 0  Threshold=double(0)  OutDataTypeStr=fixdt(0, 12, 0)  SampleTime=1e-08  SaturateOnIntegerOverflow=off  InputSameDT=off
  Out1 : Outport  OutDataTypeStr=boolean  SampleTime=1e-08
  wires:
  enb/1 -> NOT/1, switchEnable/1
  AND/1 -> Out1/1
  Constant/1 -> Switch1/1, Switch/3
  Constant1/1 -> Switch1/3, Switch/1
  Switch/1 -> AND/1
  Switch1/1 -> AND/2
  stateControl/1 -> delayMatch/1
  HDL Counter/1 -> HDL Counter_enbsw/3, adder/1, compare/1, switchEnable/2, Switch1/2, Switch/2
  delayMatch/1 -> HDL Counter_enbsw/2
  step_value/1 -> adder/2
  countFrom/1 -> switch/1
  const/1 -> switchReset/1
  NOT/1 -> switchReset/2
  adder/1 -> switch/3
  compare/1 -> switch/2
  switch/1 -> switchEnable/3
  switchEnable/1 -> switchReset/3
  switchReset/1 -> HDL Counter_enbsw/1
  HDL Counter_enbsw/1 -> HDL Counter/1

== system gm_hdl_model_fixed/Subsystem1/myRMS/CORDIC Square Root HDL Optimized ==
  u : Inport  OutDataTypeStr=fixdt(0, 16, 7)  SampleTime=1e-08
  validIn : Inport  Port=2  OutDataTypeStr=boolean  SampleTime=1e-08
  restart : Inport  Port=3  OutDataTypeStr=boolean  SampleTime=1e-08
  Bit Shift Arithmetic : Subsystem
  Cast to Union of Types : Subsystem
  Data Type Conversion : DataTypeConversion  OutDataTypeStr=fixdt(0, 16, 7)  RndMeth=Nearest  SampleTime=1e-08  SaturateOnIntegerOverflow=off
  Synchronous Subsystem : Subsystem
  y : Outport  SampleTime=1e-08
  validOut : Outport  Port=2  SampleTime=1e-08
  wires:
  u/1 -> Cast to Union of Types/1(Xref), Synchronous Subsystem/1(u)
  validIn/1 -> Synchronous Subsystem/2(validIn)
  restart/1 -> Synchronous Subsystem/3(restart)
  Bit Shift Arithmetic/1(y) -> Data Type Conversion/1
  Cast to Union of Types/1(Cout) -> Bit Shift Arithmetic/1(u)
  Data Type Conversion/1 -> y/1
  Synchronous Subsystem/1(dataOut) -> Cast to Union of Types/2(Cin)
  Synchronous Subsystem/2(eOut) -> Bit Shift Arithmetic/2(e)
  Synchronous Subsystem/3(isZero) -> Bit Shift Arithmetic/3(isZero)
  Synchronous Subsystem/4(validOut) -> validOut/1

== system gm_hdl_model_fixed/Subsystem1/myRMS/Sample and Hold ==
  In : Inport  OutDataTypeStr=fixdt(0, 16, 7)
  Trigger : TriggerPort  VariantControl=(inherit)  OutDataTypeStr=boolean
  " " : Outport  InitialOutput=0
  wires:
  In/1 -> " "/1

== system gm_hdl_model_fixed/Subsystem1/Subsystem Reference/Absolute of Complex/CORDIC Square Root HDL Optimized1 ==
  u : Inport  OutDataTypeStr=fixdt(1, 24, 22)  SampleTime=1e-08
  validIn : Inport  Port=2  OutDataTypeStr=boolean  SampleTime=1e-08
  restart : Inport  Port=3  OutDataTypeStr=boolean  SampleTime=1e-08
  Bit Shift Arithmetic : Subsystem
  Cast to Union of Types : Subsystem
  Data Type Conversion : DataTypeConversion  OutDataTypeStr=fixdt(1,24,22)
  Synchronous Subsystem : Subsystem
  y : Outport  SampleTime=1e-08
  validOut : Outport  Port=2  SampleTime=1e-08
  wires:
  u/1 -> Cast to Union of Types/1(Xref), Synchronous Subsystem/1(u)
  validIn/1 -> Synchronous Subsystem/2(validIn)
  restart/1 -> Synchronous Subsystem/3(restart)
  Bit Shift Arithmetic/1(y) -> Data Type Conversion/1
  Cast to Union of Types/1(Cout) -> Bit Shift Arithmetic/1(u)
  Data Type Conversion/1 -> y/1
  Synchronous Subsystem/1(dataOut) -> Cast to Union of Types/2(Cin)
  Synchronous Subsystem/2(eOut) -> Bit Shift Arithmetic/2(e)
  Synchronous Subsystem/3(isZero) -> Bit Shift Arithmetic/3(isZero)
  Synchronous Subsystem/4(validOut) -> validOut/1

== system gm_hdl_model_fixed/Subsystem1/Subsystem Reference/CORDIC Square Root HDL Optimized/Bit Shift Arithmetic ==
  u : Inport  OutDataTypeStr=fixdt(1, 22, 20)  PortDimensions=1  SampleTime=1e-08
  e : Inport  Port=2  OutDataTypeStr=int32  PortDimensions=1  SampleTime=1e-08
  isZero : Inport  Port=3  OutDataTypeStr=boolean  PortDimensions=1  SampleTime=1e-08
  embmathops_c6_sxviEMGenxpVSWTChSq0GHG_Bit_Shift_Arithmetic : MATLAB Function  TreatAsAtomicUnit=on
      settings: LibrarySourceBlock=embmathops/CORDIC Square Root HDL Optimized/Bit Shift Arithmetic
  y : Outport  SampleTime=1e-08  VectorParamsAs1DForOutWhenUnconnected=off
  wires:
  u/1 -> embmathops_c6_sxviEMGenxpVSWTChSq0GHG_Bit_Shift_Arithmetic/1(u)
  e/1 -> embmathops_c6_sxviEMGenxpVSWTChSq0GHG_Bit_Shift_Arithmetic/2(e)
  isZero/1 -> embmathops_c6_sxviEMGenxpVSWTChSq0GHG_Bit_Shift_Arithmetic/3(isZero)
  embmathops_c6_sxviEMGenxpVSWTChSq0GHG_Bit_Shift_Arithmetic/1(y) -> y/1

== system gm_hdl_model_fixed/Subsystem1/Subsystem Reference/CORDIC Square Root HDL Optimized/Cast to Union of Types ==
  Xref : Inport  OutDataTypeStr=fixdt(1, 22, 20)  SampleTime=1e-08
  Cin : Inport  Port=2  OutDataTypeStr=fixdt(1, 22, 20)  SampleTime=1e-08
  slutils_c1_sUkuwzpcxqKl25e4GzDa0OH_Cast_to_Union_of_Types : MATLAB Function
      settings: LibrarySourceBlock=slutils/Cast to Union of Types
  Cout : Outport  SampleTime=1e-08
  wires:
  Xref/1 -> slutils_c1_sUkuwzpcxqKl25e4GzDa0OH_Cast_to_Union_of_Types/1(Xref)
  Cin/1 -> slutils_c1_sUkuwzpcxqKl25e4GzDa0OH_Cast_to_Union_of_Types/2(Cin)
  slutils_c1_sUkuwzpcxqKl25e4GzDa0OH_Cast_to_Union_of_Types/1(Cout) -> Cout/1

== system gm_hdl_model_fixed/Subsystem1/Subsystem Reference/CORDIC Square Root HDL Optimized/Synchronous Subsystem ==
  u : Inport  OutDataTypeStr=fixdt(1, 22, 20)  PortDimensions=1  SampleTime=1e-08
  validIn : Inport  Port=2  OutDataTypeStr=boolean  PortDimensions=1  SampleTime=1e-08
  restart : Inport  Port=3  OutDataTypeStr=boolean  PortDimensions=1  SampleTime=1e-08
  StateControl : StateControl  StateControl=Synchronous
  cordicSquareRootHDL : Subsystem
  dataOut : Outport  SampleTime=1e-08  VectorParamsAs1DForOutWhenUnconnected=off
  eOut : Outport  Port=2  SampleTime=1e-08  VectorParamsAs1DForOutWhenUnconnected=off
  isZero : Outport  Port=3  SampleTime=1e-08  VectorParamsAs1DForOutWhenUnconnected=off
  validOut : Outport  Port=4  SampleTime=1e-08  VectorParamsAs1DForOutWhenUnconnected=off
  wires:
  u/1 -> cordicSquareRootHDL/1(u)
  validIn/1 -> cordicSquareRootHDL/2(validIn)
  restart/1 -> cordicSquareRootHDL/3(restart)
  cordicSquareRootHDL/1(dataOut) -> dataOut/1
  cordicSquareRootHDL/2(eOut) -> eOut/1
  cordicSquareRootHDL/3(isZero) -> isZero/1
  cordicSquareRootHDL/4(validOut) -> validOut/1
